simulink library "AIL_STATE_MACHINE_LIB"  (R2021b)
settings: Solver=VariableStepAuto  StartTime=0.0  StopTime=10.0  RelTol=1e-3
settings Model: Creator=ACH  LastModifiedBy=ACH

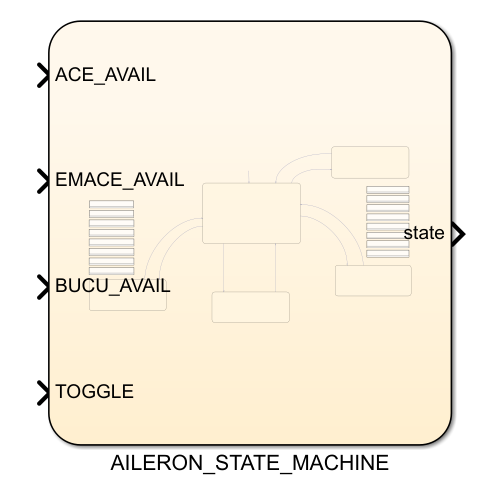
[thumbnail: Simulink's stored preview of the top-level diagram]
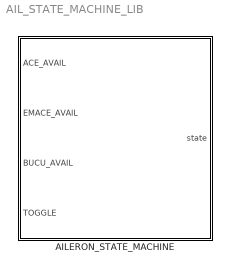
== system AIL_STATE_MACHINE_LIB ==
  AILERON_STATE_MACHINE : Stateflow chart  TreatAsAtomicUnit=on

== stateflow chart AIL_STATE_MACHINE_LIB/AILERON_STATE_MACHINE ==
  state BRAKE
    state = 4;
    %--------------------------------------------------------------------------------------------------------
    entry:
    count40 = 0;
    %--------------------------------------------------------------------------------------------------------
    during:
    cond40 = transition40(ACE_AVAIL,EMACE_AVAIL,BUCU_AVAIL,TOGGLE);
    count40 = delay40(cond40,count40);
    %--------------------------------------------------------------------------------------------------------
    exit:
    count40 = 0;
  state LOSS
    state = 0;
    %--------------------------------------------------------------------------------------------------------
    entry:
    count01 = 0;
    count02 = 0;
    count03 = 0;
    count04 = 0;
    %--------------------------------------------------------------------------------------------------------
    during:
    cond01 = transition01(ACE_AVAIL,EMACE_AVAIL,BUCU_AVAIL,TOGGLE);
    cond02 = transition02(ACE_AVAIL,EMACE_AVAIL,BUCU_AVAIL,TOGGLE);
    cond03 = transition03(ACE_AVAIL,EMACE_AVAIL,BUCU_AVAIL,TOGGLE);
    cond04 = transition04(ACE_AVAIL,EMACE_AVAIL,BUCU_AVAIL,TOGGLE);
    count01 = delay01(cond01,count01);
    count02 = delay02(cond02,count02);
    count03 = delay03(cond03,count03);
    count04 = delay04(cond04,count04);
    %--------------------------------------------------------------------------------------------------------
    exit:
    count01 = 0;
    count02 = 0;
    count03 = 0;
    count04 = 0;
  state ELECTRIC
    state = 2;
    %--------------------------------------------------------------------------------------------------------
    entry:
    count20 = 0;
    %--------------------------------------------------------------------------------------------------------
    during:
    cond20 = transition20(ACE_AVAIL,EMACE_AVAIL,BUCU_AVAIL,TOGGLE);
    count20 = delay20(cond20,count20);
    %--------------------------------------------------------------------------------------------------------
    exit:
    count20 = 0;
  state HYDRAULIC
    state = 1;
    %--------------------------------------------------------------------------------------------------------
    entry:
    count10 = 0;
    %--------------------------------------------------------------------------------------------------------
    during:
    cond10 = transition10(ACE_AVAIL,EMACE_AVAIL,BUCU_AVAIL,TOGGLE);
    count10 = delay10(cond10,count10);
    %--------------------------------------------------------------------------------------------------------
    exit:
    count10 = 0;
  state BACKUP
    state = 3;
    %--------------------------------------------------------------------------------------------------------
    entry:
    count30 = 0;
    %--------------------------------------------------------------------------------------------------------
    during:
    cond30 = transition30(ACE_AVAIL,EMACE_AVAIL,BUCU_AVAIL,TOGGLE);
    count30 = delay30(cond30,count30);
    %--------------------------------------------------------------------------------------------------------
    exit:
    count30 = 0;
  BRAKE -> LOSS : [((ACE_AVAIL== 1) | ...
      | (EMACE_AVAIL == 1) | ...
      | (BUCU_AVAIL == 1)) & ...
      | (count40 == 200)]
  LOSS -> BRAKE [order 4] : [((ACE_AVAIL == 0) &...
      | (EMACE_AVAIL == 0) &...
      | (BUCU_AVAIL == 0)) & ...
      | (count04 ==500)]
  (default) -> LOSS
  ELECTRIC -> LOSS : [((EMACE_AVAIL == 0) | ...
      | ((ACE_AVAIL == 1) & (TOGGLE == 0))) & ...
      | (count20 == 100)]
  LOSS -> ELECTRIC [order 2] : [(((EMACE_AVAIL == 1) & (TOGGLE == 1)) | ...
      | ((EMACE_AVAIL == 1) & (ACE_AVAIL == 0))) & ...
      | (count02 == 100)]
  HYDRAULIC -> LOSS : [((ACE_AVAIL == 0) | ...
      | ((ACE_AVAIL== 1) & (TOGGLE == 1) & (EMACE_AVAIL == 1))) & ...
      | (count10 == 100)]
  LOSS -> HYDRAULIC [order 1] : [(((ACE_AVAIL == 1) & (TOGGLE == 0)) | ...
      | ((EMACE_AVAIL == 0) & (ACE_AVAIL == 1))) & ...
      | (count01 == 100)]
  LOSS -> BACKUP [order 3] : [((ACE_AVAIL == 0) & ...
      | (EMACE_AVAIL == 0) & ...
      | (BUCU_AVAIL == 1)) & ...
      | (count03 == 100)]
  BACKUP -> LOSS : [((BUCU_AVAIL == 0) | ...
      | ((ACE_AVAIL == 1) | (EMACE_AVAIL == 1))) & ...
      |  (count30 == 100)]
  data: condition01 function_input; counter01 function_input; counter01 function_output; condition02 function_input; counter02 function_input; counter02 function_output; ACE function_input; EMACE function_input; BUCU function_input; TOGG function_input; tr01 function_output; condition03 function_input; counter03 function_input; counter03 function_output; ACE function_input; EMACE function_input; BUCU function_input; TOGG function_input; tr02 function_output; condition04 function_input; counter04 function_input; counter04 function_output; ACE function_input; EMACE function_input; BUCU function_input; TOGG function_input; tr03 function_output; condition10 function_input; counter10 function_input; counter10 function_output; ACE function_input; EMACE function_input; BUCU function_input; TOGG function_input; tr04 function_output; condition20 function_input; counter20 function_input; counter20 function_output; ACE function_input; EMACE function_input; BUCU function_input; TOGG function_input; tr10 function_output; condition30 function_input; counter30 function_input; counter30 function_output; ACE function_input; EMACE function_input; BUCU function_input; TOGG function_input; tr20 function_output; condition40 function_input; counter40 function_input; counter40 function_output; ACE function_input; EMACE function_input; BUCU function_input; TOGG function_input; tr30 function_output; ACE function_input; EMACE function_input; BUCU function_input; TOGG function_input; tr40 function_output; ACE_AVAIL input; EMACE_AVAIL input; BUCU_AVAIL input; TOGGLE input; state output; TOGGLE1 local; ACE_AVAIL1 local; EMACE_AVAIL1 local; BUCU_AVAIL1 local; count02 local; count01 local; count03 local; cond01 local; count30 local; cond30 local; count20 local; cond20 local; count10 local; cond10 local; cond02 local; cond03 local; cond40 local; count40 local; count04 local; cond04 local
  function counter01=delay01(condition01,counter01):
    | function counter01=delay01(condition01,counter01)
    | if (condition01 == 1)
    |     counter01 = counter01 + 1;
    | else
    |     counter01 = 0;
    | end
    | end
  function counter02=delay02(condition02,counter02):
    | function counter02=delay02(condition02,counter02)
    | if (condition02 == 1)
    |     counter02 = counter02 + 1;
    | else
    |     counter02 = 0;
    | end
    | end
  function tr01=transition01(ACE,EMACE,BUCU,TOGG):
    | function tr01=transition01(ACE,EMACE,BUCU,TOGG)
    | tr01 = (((ACE == 1) & (TOGG == 0)) | ((EMACE == 0) & (ACE == 1)));
    | % tr02 = ((EMACE == 1) & (TOGG == 1)) | ((EMACE == 1) & (ACE == 0));
    | % tr03 = ((ACE == 0) & (EMACE == 0) & (BUCU == 1));
    | % tr10 = ((ACE == 0) | ((ACE == 1) & (TOGG == 1) & (EMACE == 1)));
    | % tr20 = ((EMACE == 0) | ((ACE == 1) & (TOGG == 0)));
    | % tr30 =  ((BUCU == 0) | (ACE == 1) | (EMACE == 1));
    | end
  function counter03=delay03(condition03,counter03):
    | function counter03=delay03(condition03,counter03)
    | if (condition03 == 1)
    |     counter03 = counter03 + 1;
    | else
    |     counter03 = 0;
    | end
    | end
  function tr02=transition02(ACE,EMACE,BUCU,TOGG):
    | function tr02=transition02(ACE,EMACE,BUCU,TOGG)
    | % tr01 = (((ACE == 1) & (TOGG == 0)) | ((EMACE == 0) & (ACE == 1)));
    | tr02 = ((EMACE == 1) & (TOGG == 1)) | ((EMACE == 1) & (ACE == 0));
    | % tr03 = ((ACE == 0) & (EMACE == 0) & (BUCU == 1));
    | % tr10 = ((ACE == 0) | ((ACE == 1) & (TOGG == 1) & (EMACE == 1)));
    | % tr20 = ((EMACE == 0) | ((ACE == 1) & (TOGG == 0)));
    | % tr30 =  ((BUCU == 0) | (ACE == 1) | (EMACE == 1));
    | end
  function counter04=delay04(condition04,counter04):
    | function counter04=delay04(condition04,counter04)
    | if (condition04 == 1)
    |     counter04 = counter04 + 1;
    | else
    |     counter04 = 0;
    | end
    | end
  function tr03=transition03(ACE,EMACE,BUCU,TOGG):
    | function tr03=transition03(ACE,EMACE,BUCU,TOGG)
    | % tr01 = (((ACE == 1) & (TOGG == 0)) | ((EMACE == 0) & (ACE == 1)));
    | % tr02 = ((EMACE == 1) & (TOGG == 1)) | ((EMACE == 1) & (ACE == 0));
    | tr03 = ((ACE == 0) & (EMACE == 0) & (BUCU == 1));
    | % tr10 = ((ACE == 0) | ((ACE == 1) & (TOGG == 1) & (EMACE == 1)));
    | % tr20 = ((EMACE == 0) | ((ACE == 1) & (TOGG == 0)));
    | % tr30 =  ((BUCU == 0) | (ACE == 1) | (EMACE == 1));
    | end
  function counter10=delay10(condition10,counter10):
    | function counter10=delay10(condition10,counter10)
    | if (condition10 == 1)
    |     counter10 = counter10 + 1;
    | else
    |     counter10 = 0;
    | end
    | end
  function tr04=transition04(ACE,EMACE,BUCU,TOGG):
    | function tr04=transition04(ACE,EMACE,BUCU,TOGG)
    | % tr01 = (((ACE == 1) & (TOGG == 0)) | ((EMACE == 0) & (ACE == 1)));
    | % tr02 = ((EMACE == 1) & (TOGG == 1)) | ((EMACE == 1) & (ACE == 0));
    | % tr03 = ((ACE == 0) & (EMACE == 0) & (BUCU == 1));
    | tr04 = ((ACE == 0) & (EMACE == 0) & (BUCU == 0));
    | % tr10 = ((ACE == 0) | ((ACE == 1) & (TOGG == 1) & (EMACE == 1)));
    | % tr20 = ((EMACE == 0) | ((ACE == 1) & (TOGG == 0)));
    | % tr30 =  ((BUCU == 0) | (ACE == 1) | (EMACE == 1));
    | end
  function counter20=delay20(condition20,counter20):
    | function counter20=delay20(condition20,counter20)
    | if (condition20 == 1)
    |     counter20 = counter20 + 1;
    | else
    |     counter20 = 0;
    | end
    | end
  function tr10=transition10(ACE,EMACE,BUCU,TOGG):
    | function tr10=transition10(ACE,EMACE,BUCU,TOGG)
    | % tr01 = (((ACE == 1) & (TOGG == 0)) | ((EMACE == 0) & (ACE == 1)));
    | % tr02 = ((EMACE == 1) & (TOGG == 1)) | ((EMACE == 1) & (ACE == 0));
    | % tr03 = ((ACE == 0) & (EMACE == 0) & (BUCU == 1));
    | tr10 = ((ACE == 0) | ((ACE == 1) & (TOGG == 1) & (EMACE == 1)));
    | % tr20 = ((EMACE == 0) | ((ACE == 1) & (TOGG == 0)));
    | % tr30 =  ((BUCU == 0) | (ACE == 1) | (EMACE == 1));
    | end
  function counter30=delay30(condition30,counter30):
    | function counter30=delay30(condition30,counter30)
    | if (condition30 == 1)
    |     counter30 = counter30 + 1;
    | else
    |     counter30 = 0;
    | end
    | end
  function tr20=transition20(ACE,EMACE,BUCU,TOGG):
    | function tr20=transition20(ACE,EMACE,BUCU,TOGG)
    | % tr01 = (((ACE == 1) & (TOGG == 0)) | ((EMACE == 0) & (ACE == 1)));
    | % tr02 = ((EMACE == 1) & (TOGG == 1)) | ((EMACE == 1) & (ACE == 0));
    | % tr03 = ((ACE == 0) & (EMACE == 0) & (BUCU == 1));
    | % tr10 = ((ACE == 0) | ((ACE == 1) & (TOGG == 1) & (EMACE == 1)));
    | tr20 = ((EMACE == 0) | ((ACE == 1) & (TOGG == 0)));
    | % tr30 =  ((BUCU == 0) | (ACE == 1) | (EMACE == 1));
    | end
  function counter40=delay40(condition40,counter40):
    | function counter40=delay40(condition40,counter40)
    | if (condition40 == 1)
    |     counter40 = counter40 + 1;
    | else
    |     counter40 = 0;
    | end
    | end
  function tr30=transition30(ACE,EMACE,BUCU,TOGG):
    | function tr30=transition30(ACE,EMACE,BUCU,TOGG)
    | % tr01 = (((ACE == 1) & (TOGG == 0)) | ((EMACE == 0) & (ACE == 1)));
    | % tr02 = ((EMACE == 1) & (TOGG == 1)) | ((EMACE == 1) & (ACE == 0));
    | % tr03 = ((ACE == 0) & (EMACE == 0) & (BUCU == 1));
    | % tr10 = ((ACE == 0) | ((ACE == 1) & (TOGG == 1) & (EMACE == 1)));
    | % tr20 = ((EMACE == 0) | ((ACE == 1) & (TOGG == 0)));
    | tr30 =  ((BUCU == 0) | (ACE == 1) | (EMACE == 1));
    | end
  function tr40=transition40(ACE,EMACE,BUCU,TOGG):
    | function tr40=transition40(ACE,EMACE,BUCU,TOGG)
    | % tr01 = (((ACE == 1) & (TOGG == 0)) | ((EMACE == 0) & (ACE == 1)));
    | % tr02 = ((EMACE == 1) & (TOGG == 1)) | ((EMACE == 1) & (ACE == 0));
    | % tr03 = ((ACE == 0) & (EMACE == 0) & (BUCU == 1));
    | % tr10 = ((ACE == 0) | ((ACE == 1) & (TOGG == 1) & (EMACE == 1)));
    | % tr20 = ((EMACE == 0) | ((ACE == 1) & (TOGG == 0)));
    | % tr30 =  ((BUCU == 0) | (ACE == 1) | (EMACE == 1));
    | tr40 = ((ACE == 1) | (EMACE == 1) | (BUCU == 1));
    | end
